simulink model "model_sim_CHB5_36_new_temp"  (R2020a)
settings: Solver=FixedStepAuto  StartTime=0.0  StopTime=5  RelTol=1e-3
InitFcn:
  | sysinit
values from neighbouring files (symbols this model uses):
  C = 0.03    [sysinit.m]
  C_f = 0.625e-6    (= 6.25e-07)    [sysinit.m]
  f = 50    [sysinit.m]
  f_switch = 500    [sysinit.m]
  L = 0.004    [sysinit.m]
  L_f = 3e-6    (= 3e-06)    [sysinit.m]
  R = 1.2    [sysinit.m]
  R_f = 1.5    [sysinit.m]
  Rth_h = 7.5e-3    (= 0.0075)    [Device_Parameter.m]
  Rth_h_tau = 0.5    [Device_Parameter.m]
  st = 5e-7    (= 5e-07)    [sysinit.m]
  temp_init = 40    [sysinit.m]
  Ts = 1e-6    (= 1e-06)    [sysinit.m]
  Ts2 = 0.5E-3    (= 0.0005)    [sysinit.m]
  Udc = 2500    [sysinit.m]
undefined symbols (not defined in the file or in its folder): DIODE_204520, DIODE_344520, DIODE_D1031SH, DIODE_D1331SH, IGCT_364520_36, IGCT_364521_36, IGCT_654522_6, magnitude, Ts1
libraries: powerlib x278, powerlib_meascontrol x84, simulink x9
(part 3 of 5)

== system model_sim_CHB5_36_new_temp/Uref/Saddle_Wave ==
  A : Inport
  B : Inport  Port=2
  C : Inport  Port=3
  Add{1..3,9} (4 alike) : Sum
  Gain : Gain  Gain=-0.5
  Max : MinMax  Function=max  Inputs=3
  Max1 : MinMax  Inputs=3
  a : Outport
  b : Outport  Port=2
  c : Outport  Port=3
  wires:
  B/1 -> Add3/2, Max1/2, Max/2
  C/1 -> Add9/2, Max1/3, Max/3
  A/1 -> Max1/1, Add2/2, Max/1
  Gain/1 -> Add9/1, Add3/1, Add2/1
  Max/1 -> Add1/1
  Max1/1 -> Add1/2
  Add1/1 -> Gain/1
  Add9/1 -> c/1
  Add2/1 -> a/1
  Add3/1 -> b/1

== system model_sim_CHB5_36_new_temp/pwm generator/carrier ==
  Mux : Mux
  Repeating Sequence1 : simulink/Sources/Repeating Sequence  rep_seq_t=[0 0.5 1]/f_car  rep_seq_y=[-1 1 -1]*1000
  Scope1 : Scope  NumInputPorts=4
  Transport Delay1 : TransportDelay  DelayTime=tt/f_car  BufferSize=3072
  Transport Delay3 : TransportDelay  DelayTime=tt/f_car  BufferSize=3072
  Transport Delay4 : TransportDelay  DelayTime=tt/f_car  BufferSize=3072
  CARRIER_4*1 : Outport
  wires:
  Repeating Sequence1/1 -> Scope1/1, Mux/1, Transport Delay1/1
  Transport Delay1/1 -> Scope1/2, Mux/2, Transport Delay3/1
  Mux/1 -> CARRIER_4*1/1
  Transport Delay3/1 -> Mux/3, Scope1/3, Transport Delay4/1
  Transport Delay4/1 -> Mux/4, Scope1/4

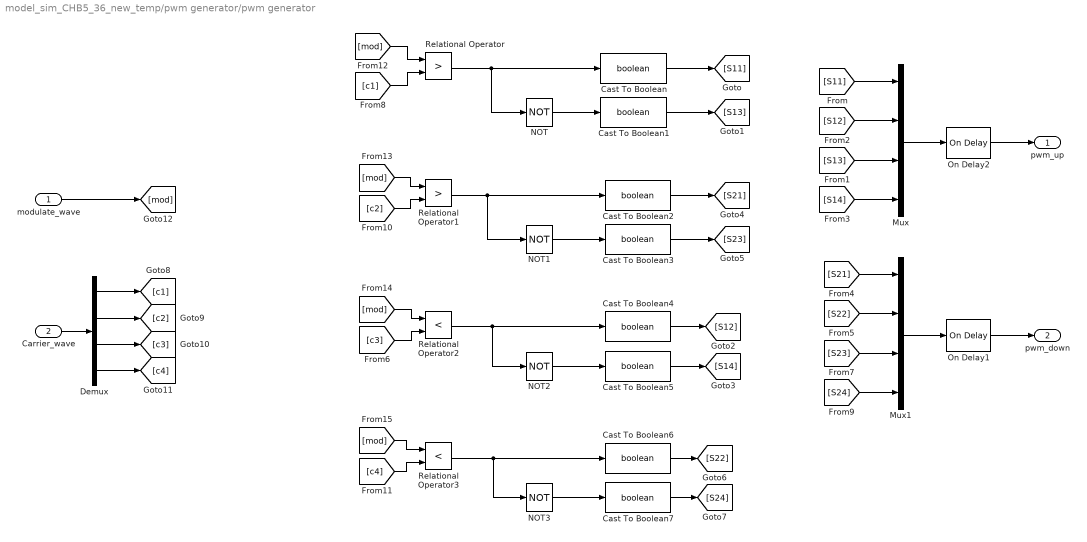
== system model_sim_CHB5_36_new_temp/pwm generator/pwm generator ==
  modulate_wave : Inport
  Carrier_wave : Inport  Port=2
  Cast To Boolean{,1..7} (8 alike) : DataTypeConversion  OutDataTypeStr=boolean
  Demux : Demux
  Mux : Mux
  Mux1 : Mux
  NOT{,1..3} (4 alike) : Logic  Operator=NOT  AllPortsSameDT=off  OutDataTypeStr=boolean
  On Delay1 : powerlib_meascontrol/Logic/On Delay  DelayType=On delay  delay=ttd  ic=0  Ts=0
  On Delay2 : powerlib_meascontrol/Logic/On Delay  DelayType=On delay  delay=ttd  ic=0  Ts=0
  Relational Operator : RelationalOperator  Operator=>  OutDataTypeStr=boolean  RndMeth=Simplest
  Relational Operator1 : RelationalOperator  Operator=>  OutDataTypeStr=boolean  RndMeth=Simplest
  Relational Operator2 : RelationalOperator  Operator=<  OutDataTypeStr=boolean  RndMeth=Simplest
  Relational Operator3 : RelationalOperator  Operator=<  OutDataTypeStr=boolean  RndMeth=Simplest
  pwm_up : Outport
  pwm_down : Outport  Port=2
  wires:
  NOT/1 -> Cast To Boolean1/1
  [S14] -> Mux/4
  [S23] -> Mux1/3
  [S12] -> Mux/2
  NOT2/1 -> Cast To Boolean5/1
  [S21] -> Mux1/1
  Relational Operator1/1 -> NOT1/1, Cast To Boolean2/1
  [S22] -> Mux1/2
  NOT3/1 -> Cast To Boolean7/1
  Mux/1 -> On Delay2/1
  [S24] -> Mux1/4
  [S13] -> Mux/3
  Relational Operator2/1 -> Cast To Boolean4/1, NOT2/1
  [S11] -> Mux/1
  Relational Operator/1 -> NOT/1, Cast To Boolean/1
  NOT1/1 -> Cast To Boolean3/1
  Mux1/1 -> On Delay1/1
  Relational Operator3/1 -> Cast To Boolean6/1, NOT3/1
  On Delay1/1 -> pwm_down/1
  On Delay2/1 -> pwm_up/1
  Cast To Boolean/1 -> [S11]
  Cast To Boolean1/1 -> [S13]
  Cast To Boolean2/1 -> [S21]
  Cast To Boolean3/1 -> [S23]
  Cast To Boolean4/1 -> [S12]
  Cast To Boolean5/1 -> [S14]
  Cast To Boolean6/1 -> [S22]
  Cast To Boolean7/1 -> [S24]
  Carrier_wave/1 -> Demux/1
  Demux/1 -> [c1]
  [c3] -> Relational Operator2/2
  Demux/2 -> [c2]
  Demux/4 -> [c4]
  Demux/3 -> [c3]
  [c1] -> Relational Operator/2
  [c2] -> Relational Operator1/2
  [c4] -> Relational Operator3/2
  modulate_wave/1 -> [mod]
  [mod] -> Relational Operator/1
  [mod] -> Relational Operator3/1
  [mod] -> Relational Operator2/1
  [mod] -> Relational Operator1/1

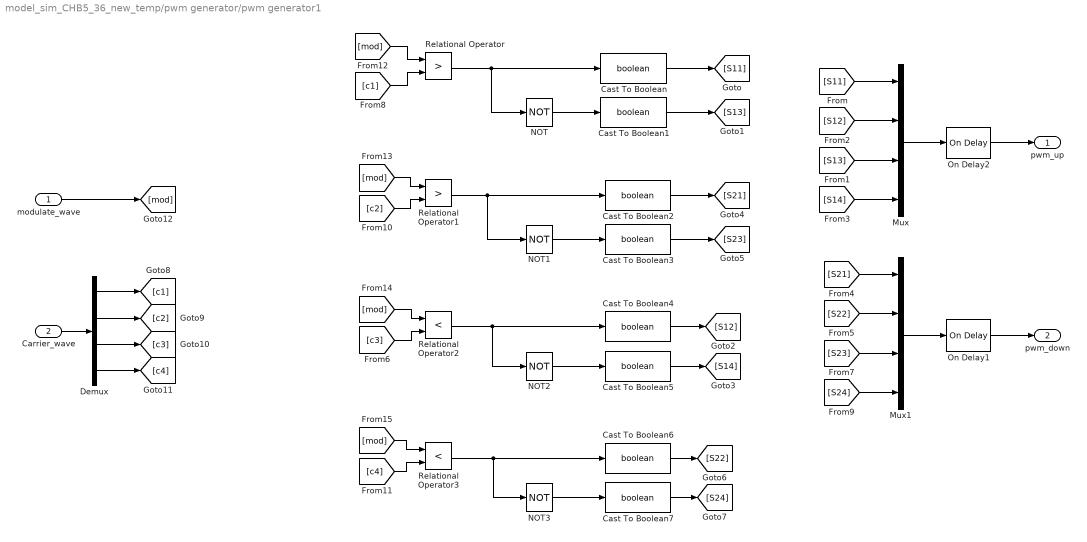
== system model_sim_CHB5_36_new_temp/pwm generator/pwm generator1 ==
  modulate_wave : Inport
  Carrier_wave : Inport  Port=2
  Cast To Boolean{,1..7} (8 alike) : DataTypeConversion  OutDataTypeStr=boolean
  Demux : Demux
  Mux : Mux
  Mux1 : Mux
  NOT{,1..3} (4 alike) : Logic  Operator=NOT  AllPortsSameDT=off  OutDataTypeStr=boolean
  On Delay1 : powerlib_meascontrol/Logic/On Delay  DelayType=On delay  delay=ttd  ic=0  Ts=0
  On Delay2 : powerlib_meascontrol/Logic/On Delay  DelayType=On delay  delay=ttd  ic=0  Ts=0
  Relational Operator : RelationalOperator  Operator=>  OutDataTypeStr=boolean  RndMeth=Simplest
  Relational Operator1 : RelationalOperator  Operator=>  OutDataTypeStr=boolean  RndMeth=Simplest
  Relational Operator2 : RelationalOperator  Operator=<  OutDataTypeStr=boolean  RndMeth=Simplest
  Relational Operator3 : RelationalOperator  Operator=<  OutDataTypeStr=boolean  RndMeth=Simplest
  pwm_up : Outport
  pwm_down : Outport  Port=2
  wires:
  [mod] -> Relational Operator1/1
  [mod] -> Relational Operator2/1
  [mod] -> Relational Operator3/1
  [mod] -> Relational Operator/1
  modulate_wave/1 -> [mod]
  [c4] -> Relational Operator3/2
  [c2] -> Relational Operator1/2
  [c1] -> Relational Operator/2
  Demux/3 -> [c3]
  Demux/4 -> [c4]
  Demux/2 -> [c2]
  [c3] -> Relational Operator2/2
  Demux/1 -> [c1]
  Carrier_wave/1 -> Demux/1
  Cast To Boolean7/1 -> [S24]
  Cast To Boolean6/1 -> [S22]
  Cast To Boolean5/1 -> [S14]
  Cast To Boolean4/1 -> [S12]
  Cast To Boolean3/1 -> [S23]
  Cast To Boolean2/1 -> [S21]
  Cast To Boolean1/1 -> [S13]
  Cast To Boolean/1 -> [S11]
  On Delay2/1 -> pwm_up/1
  On Delay1/1 -> pwm_down/1
  Relational Operator3/1 -> NOT3/1, Cast To Boolean6/1
  Mux1/1 -> On Delay1/1
  NOT1/1 -> Cast To Boolean3/1
  Relational Operator/1 -> Cast To Boolean/1, NOT/1
  [S11] -> Mux/1
  Relational Operator2/1 -> NOT2/1, Cast To Boolean4/1
  [S13] -> Mux/3
  [S24] -> Mux1/4
  Mux/1 -> On Delay2/1
  NOT3/1 -> Cast To Boolean7/1
  [S22] -> Mux1/2
  Relational Operator1/1 -> Cast To Boolean2/1, NOT1/1
  [S21] -> Mux1/1
  NOT2/1 -> Cast To Boolean5/1
  [S12] -> Mux/2
  [S23] -> Mux1/3
  [S14] -> Mux/4
  NOT/1 -> Cast To Boolean1/1

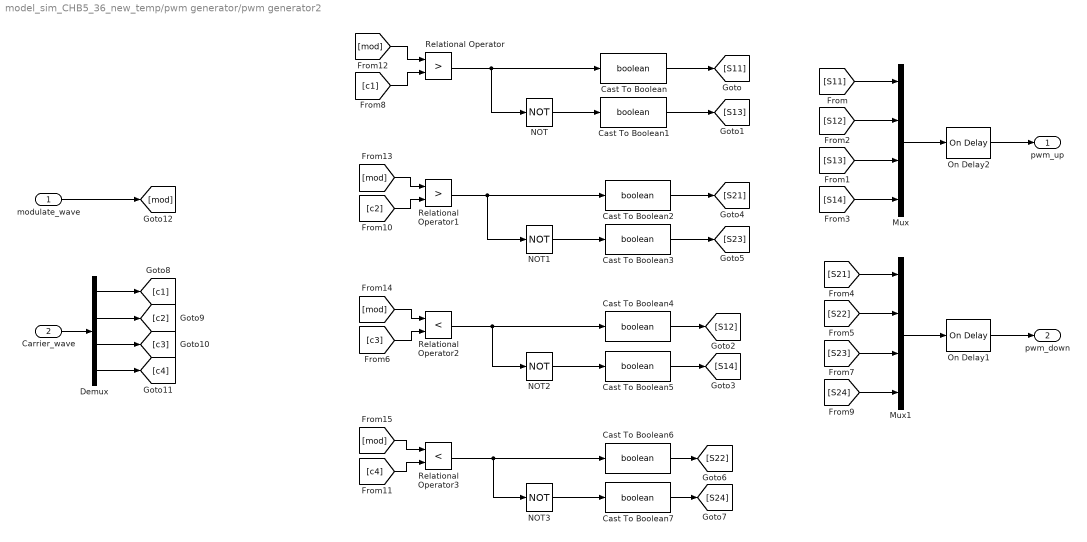
== system model_sim_CHB5_36_new_temp/pwm generator/pwm generator2 ==
  modulate_wave : Inport
  Carrier_wave : Inport  Port=2
  Cast To Boolean{,1..7} (8 alike) : DataTypeConversion  OutDataTypeStr=boolean
  Demux : Demux
  Mux : Mux
  Mux1 : Mux
  NOT{,1..3} (4 alike) : Logic  Operator=NOT  AllPortsSameDT=off  OutDataTypeStr=boolean
  On Delay1 : powerlib_meascontrol/Logic/On Delay  DelayType=On delay  delay=ttd  ic=0  Ts=0
  On Delay2 : powerlib_meascontrol/Logic/On Delay  DelayType=On delay  delay=ttd  ic=0  Ts=0
  Relational Operator : RelationalOperator  Operator=>  OutDataTypeStr=boolean  RndMeth=Simplest
  Relational Operator1 : RelationalOperator  Operator=>  OutDataTypeStr=boolean  RndMeth=Simplest
  Relational Operator2 : RelationalOperator  Operator=<  OutDataTypeStr=boolean  RndMeth=Simplest
  Relational Operator3 : RelationalOperator  Operator=<  OutDataTypeStr=boolean  RndMeth=Simplest
  pwm_up : Outport
  pwm_down : Outport  Port=2
  wires:
  NOT/1 -> Cast To Boolean1/1
  [S14] -> Mux/4
  [S23] -> Mux1/3
  [S12] -> Mux/2
  NOT2/1 -> Cast To Boolean5/1
  [S21] -> Mux1/1
  Relational Operator1/1 -> NOT1/1, Cast To Boolean2/1
  [S22] -> Mux1/2
  NOT3/1 -> Cast To Boolean7/1
  Mux/1 -> On Delay2/1
  [S24] -> Mux1/4
  [S13] -> Mux/3
  Relational Operator2/1 -> Cast To Boolean4/1, NOT2/1
  [S11] -> Mux/1
  Relational Operator/1 -> NOT/1, Cast To Boolean/1
  NOT1/1 -> Cast To Boolean3/1
  Mux1/1 -> On Delay1/1
  Relational Operator3/1 -> Cast To Boolean6/1, NOT3/1
  On Delay1/1 -> pwm_down/1
  On Delay2/1 -> pwm_up/1
  Cast To Boolean/1 -> [S11]
  Cast To Boolean1/1 -> [S13]
  Cast To Boolean2/1 -> [S21]
  Cast To Boolean3/1 -> [S23]
  Cast To Boolean4/1 -> [S12]
  Cast To Boolean5/1 -> [S14]
  Cast To Boolean6/1 -> [S22]
  Cast To Boolean7/1 -> [S24]
  Carrier_wave/1 -> Demux/1
  Demux/1 -> [c1]
  [c3] -> Relational Operator2/2
  Demux/2 -> [c2]
  Demux/4 -> [c4]
  Demux/3 -> [c3]
  [c1] -> Relational Operator/2
  [c2] -> Relational Operator1/2
  [c4] -> Relational Operator3/2
  modulate_wave/1 -> [mod]
  [mod] -> Relational Operator/1
  [mod] -> Relational Operator3/1
  [mod] -> Relational Operator2/1
  [mod] -> Relational Operator1/1

== system model_sim_CHB5_36_new_temp/Subsystem3/DIODE/DIODE_204520 ==
  I : Inport
  PWM1 : Inport  Port=2
  PWM2 : Inport  Port=3
  PWM3 : Inport  Port=4
  PWM4 : Inport  Port=5
  Bus Creator : BusCreator  Inputs=7
  Bus Creator1 : BusCreator  Inputs=7
  Bus Selector : BusSelector  OutputSignals=D1_TEMP,D1_LOSS_MEAN
  Bus Selector1 : BusSelector  OutputSignals=D2_TEMP,D2_LOSS_MEAN
  Constant : Constant
  Constant4 : Constant  Value=0
  Constant5 : Constant
  Constant6 : Constant  Value=0
  Logical Operator : Logic  Operator=OR  AllPortsSameDT=off  OutDataTypeStr=boolean
  Subsystem5 : Subsystem
  Switch : Switch  Criteria=u2 > Threshold  Threshold=DIODE.Junc_temp_lim
  Switch1 : Switch  Criteria=u2 > Threshold  Threshold=DIODE.Junc_temp_lim
  D1_BUS : Outport
  D2_BUS : Outport  Port=2
  D1_LOSS_MEAN : Outport  Port=3
  D2_LOSS_MEAN : Outport  Port=4
  D1_TEMP : Outport  Port=5
  D2_TEMP : Outport  Port=6
  TEMLIM_BOOL : Outport  Port=7
  wires:
  I/1 -> Subsystem5/1(I)
  PWM2/1 -> Subsystem5/3(PWM2)
  PWM3/1 -> Subsystem5/4(PWM3)
  Subsystem5/3(D1_LOSS_MEAN) -> Bus Creator/3
  Subsystem5/12(D2_AVG_MEAN) -> Bus Creator1/5
  Constant6/1 -> Switch1/3
  Subsystem5/14(D2_SW_MEAN) -> Bus Creator1/7
  Switch1/1 -> Logical Operator/2
  Bus Selector1/1 -> Switch1/2, D2_TEMP/1  "<D2_TEMP>"
  Subsystem5/13(D2_SW) -> Bus Creator1/6
  Subsystem5/11(D2_AVG) -> Bus Creator1/4
  Subsystem5/8(D2_TEMP) -> Bus Creator1/1
  Subsystem5/9(D2_LOSS) -> Bus Creator1/2
  Subsystem5/7(D1_SW_MEAN) -> Bus Creator/7
  Switch/1 -> Logical Operator/1
  Constant5/1 -> Switch1/1
  Constant4/1 -> Switch/3
  Subsystem5/1(D1_TEMP) -> Bus Creator/1
  Bus Selector/1 -> Switch/2, D1_TEMP/1  "<D1_TEMP>"
  Subsystem5/6(D1_SW) -> Bus Creator/6
  Bus Creator1/1 -> [D2], D2_BUS/1  "D2_BUS"
  Subsystem5/2(D1_LOSS) -> Bus Creator/2
  Logical Operator/1 -> TEMLIM_BOOL/1
  [D1] -> Bus Selector/1
  Bus Selector/2 -> D1_LOSS_MEAN/1  "<D1_LOSS_MEAN>"
  Subsystem5/5(D1_AVG_MEAN) -> Bus Creator/5
  PWM1/1 -> Subsystem5/2(PWM1)
  PWM4/1 -> Subsystem5/5(PWM4)
  Subsystem5/4(D1_AVG) -> Bus Creator/4
  [D2] -> Bus Selector1/1
  Bus Creator/1 -> [D1], D1_BUS/1  "D1_BUS"
  Bus Selector1/2 -> D2_LOSS_MEAN/1  "<D2_LOSS_MEAN>"
  Subsystem5/10(D2_LOSS_MEAN) -> Bus Creator1/3
  Constant/1 -> Switch/1

== system model_sim_CHB5_36_new_temp/Subsystem3/DIODE/DIODE_344520 ==
  I : Inport
  PWM1 : Inport  Port=2
  PWM2 : Inport  Port=3
  PWM3 : Inport  Port=4
  PWM4 : Inport  Port=5
  Bus Creator : BusCreator  Inputs=7
  Bus Creator1 : BusCreator  Inputs=7
  Bus Selector : BusSelector  OutputSignals=D1_TEMP,D1_LOSS_MEAN
  Bus Selector1 : BusSelector  OutputSignals=D2_TEMP,D2_LOSS_MEAN
  Constant : Constant
  Constant4 : Constant  Value=0
  Constant5 : Constant
  Constant6 : Constant  Value=0
  Logical Operator : Logic  Operator=OR  AllPortsSameDT=off  OutDataTypeStr=boolean
  Subsystem5 : Subsystem
  Switch : Switch  Criteria=u2 > Threshold  Threshold=DIODE.Junc_temp_lim
  Switch1 : Switch  Criteria=u2 > Threshold  Threshold=DIODE.Junc_temp_lim
  D1_BUS : Outport
  D2_BUS : Outport  Port=2
  D1_LOSS_MEAN : Outport  Port=3
  D2_LOSS_MEAN : Outport  Port=4
  D1_TEMP : Outport  Port=5
  D2_TEMP : Outport  Port=6
  TEMLIM_BOOL : Outport  Port=7
  wires:
  Constant/1 -> Switch/1
  Subsystem5/10(D2_LOSS_MEAN) -> Bus Creator1/3
  Bus Selector1/2 -> D2_LOSS_MEAN/1  "<D2_LOSS_MEAN>"
  Bus Creator/1 -> D1_BUS/1, [D1]  "D1_BUS"
  [D2] -> Bus Selector1/1
  Subsystem5/4(D1_AVG) -> Bus Creator/4
  PWM4/1 -> Subsystem5/5(PWM4)
  PWM1/1 -> Subsystem5/2(PWM1)
  Subsystem5/5(D1_AVG_MEAN) -> Bus Creator/5
  Bus Selector/2 -> D1_LOSS_MEAN/1  "<D1_LOSS_MEAN>"
  [D1] -> Bus Selector/1
  Logical Operator/1 -> TEMLIM_BOOL/1
  Subsystem5/2(D1_LOSS) -> Bus Creator/2
  Bus Creator1/1 -> D2_BUS/1, [D2]  "D2_BUS"
  Subsystem5/6(D1_SW) -> Bus Creator/6
  Bus Selector/1 -> D1_TEMP/1, Switch/2  "<D1_TEMP>"
  Subsystem5/1(D1_TEMP) -> Bus Creator/1
  Constant4/1 -> Switch/3
  Constant5/1 -> Switch1/1
  Switch/1 -> Logical Operator/1
  Subsystem5/7(D1_SW_MEAN) -> Bus Creator/7
  Subsystem5/9(D2_LOSS) -> Bus Creator1/2
  Subsystem5/8(D2_TEMP) -> Bus Creator1/1
  Subsystem5/11(D2_AVG) -> Bus Creator1/4
  Subsystem5/13(D2_SW) -> Bus Creator1/6
  Bus Selector1/1 -> D2_TEMP/1, Switch1/2  "<D2_TEMP>"
  Switch1/1 -> Logical Operator/2
  Subsystem5/14(D2_SW_MEAN) -> Bus Creator1/7
  Constant6/1 -> Switch1/3
  Subsystem5/12(D2_AVG_MEAN) -> Bus Creator1/5
  Subsystem5/3(D1_LOSS_MEAN) -> Bus Creator/3
  PWM3/1 -> Subsystem5/4(PWM3)
  PWM2/1 -> Subsystem5/3(PWM2)
  I/1 -> Subsystem5/1(I)

== system model_sim_CHB5_36_new_temp/Subsystem3/DIODE/DIODE_D1031SH ==
  I : Inport
  PWM1 : Inport  Port=2
  PWM2 : Inport  Port=3
  PWM3 : Inport  Port=4
  PWM4 : Inport  Port=5
  Bus Creator : BusCreator  Inputs=7
  Bus Creator1 : BusCreator  Inputs=7
  Bus Selector : BusSelector  OutputSignals=D1_TEMP,D1_LOSS_MEAN
  Bus Selector1 : BusSelector  OutputSignals=D2_TEMP,D2_LOSS_MEAN
  Constant : Constant
  Constant4 : Constant  Value=0
  Constant5 : Constant
  Constant6 : Constant  Value=0
  Logical Operator : Logic  Operator=OR  AllPortsSameDT=off  OutDataTypeStr=boolean
  Subsystem5 : Subsystem
  Switch : Switch  Criteria=u2 > Threshold  Threshold=DIODE.Junc_temp_lim
  Switch1 : Switch  Criteria=u2 > Threshold  Threshold=DIODE.Junc_temp_lim
  D1_BUS : Outport
  D2_BUS : Outport  Port=2
  D1_LOSS_MEAN : Outport  Port=3
  D2_LOSS_MEAN : Outport  Port=4
  D1_TEMP : Outport  Port=5
  D2_TEMP : Outport  Port=6
  TEMLIM_BOOL : Outport  Port=7
  wires:
  I/1 -> Subsystem5/1(I)
  PWM2/1 -> Subsystem5/3(PWM2)
  PWM3/1 -> Subsystem5/4(PWM3)
  Subsystem5/3(D1_LOSS_MEAN) -> Bus Creator/3
  Subsystem5/12(D2_AVG_MEAN) -> Bus Creator1/5
  Constant6/1 -> Switch1/3
  Subsystem5/14(D2_SW_MEAN) -> Bus Creator1/7
  Switch1/1 -> Logical Operator/2
  Bus Selector1/1 -> Switch1/2, D2_TEMP/1  "<D2_TEMP>"
  Subsystem5/13(D2_SW) -> Bus Creator1/6
  Subsystem5/11(D2_AVG) -> Bus Creator1/4
  Subsystem5/8(D2_TEMP) -> Bus Creator1/1
  Subsystem5/9(D2_LOSS) -> Bus Creator1/2
  Subsystem5/7(D1_SW_MEAN) -> Bus Creator/7
  Switch/1 -> Logical Operator/1
  Constant5/1 -> Switch1/1
  Constant4/1 -> Switch/3
  Subsystem5/1(D1_TEMP) -> Bus Creator/1
  Bus Selector/1 -> Switch/2, D1_TEMP/1  "<D1_TEMP>"
  Subsystem5/6(D1_SW) -> Bus Creator/6
  Bus Creator1/1 -> [D2], D2_BUS/1  "D2_BUS"
  Subsystem5/2(D1_LOSS) -> Bus Creator/2
  Logical Operator/1 -> TEMLIM_BOOL/1
  [D1] -> Bus Selector/1
  Bus Selector/2 -> D1_LOSS_MEAN/1  "<D1_LOSS_MEAN>"
  Subsystem5/5(D1_AVG_MEAN) -> Bus Creator/5
  PWM1/1 -> Subsystem5/2(PWM1)
  PWM4/1 -> Subsystem5/5(PWM4)
  Subsystem5/4(D1_AVG) -> Bus Creator/4
  [D2] -> Bus Selector1/1
  Bus Creator/1 -> [D1], D1_BUS/1  "D1_BUS"
  Bus Selector1/2 -> D2_LOSS_MEAN/1  "<D2_LOSS_MEAN>"
  Subsystem5/10(D2_LOSS_MEAN) -> Bus Creator1/3
  Constant/1 -> Switch/1

== system model_sim_CHB5_36_new_temp/Subsystem3/DIODE/DIODE_D1331SH ==
  I : Inport
  PWM1 : Inport  Port=2
  PWM2 : Inport  Port=3
  PWM3 : Inport  Port=4
  PWM4 : Inport  Port=5
  Bus Creator : BusCreator  Inputs=7
  Bus Creator1 : BusCreator  Inputs=7
  Bus Selector : BusSelector  OutputSignals=D1_TEMP,D1_LOSS_MEAN
  Bus Selector1 : BusSelector  OutputSignals=D2_TEMP,D2_LOSS_MEAN
  Constant : Constant
  Constant4 : Constant  Value=0
  Constant5 : Constant
  Constant6 : Constant  Value=0
  Logical Operator : Logic  Operator=OR  AllPortsSameDT=off  OutDataTypeStr=boolean
  Subsystem5 : Subsystem
  Switch : Switch  Criteria=u2 > Threshold  Threshold=DIODE.Junc_temp_lim
  Switch1 : Switch  Criteria=u2 > Threshold  Threshold=DIODE.Junc_temp_lim
  D1_BUS : Outport
  D2_BUS : Outport  Port=2
  D1_LOSS_MEAN : Outport  Port=3
  D2_LOSS_MEAN : Outport  Port=4
  D1_TEMP : Outport  Port=5
  D2_TEMP : Outport  Port=6
  TEMLIM_BOOL : Outport  Port=7
  wires:
  Constant/1 -> Switch/1
  Subsystem5/10(D2_LOSS_MEAN) -> Bus Creator1/3
  Bus Selector1/2 -> D2_LOSS_MEAN/1  "<D2_LOSS_MEAN>"
  Bus Creator/1 -> D1_BUS/1, [D1]  "D1_BUS"
  [D2] -> Bus Selector1/1
  Subsystem5/4(D1_AVG) -> Bus Creator/4
  PWM4/1 -> Subsystem5/5(PWM4)
  PWM1/1 -> Subsystem5/2(PWM1)
  Subsystem5/5(D1_AVG_MEAN) -> Bus Creator/5
  Bus Selector/2 -> D1_LOSS_MEAN/1  "<D1_LOSS_MEAN>"
  [D1] -> Bus Selector/1
  Logical Operator/1 -> TEMLIM_BOOL/1
  Subsystem5/2(D1_LOSS) -> Bus Creator/2
  Bus Creator1/1 -> D2_BUS/1, [D2]  "D2_BUS"
  Subsystem5/6(D1_SW) -> Bus Creator/6
  Bus Selector/1 -> D1_TEMP/1, Switch/2  "<D1_TEMP>"
  Subsystem5/1(D1_TEMP) -> Bus Creator/1
  Constant4/1 -> Switch/3
  Constant5/1 -> Switch1/1
  Switch/1 -> Logical Operator/1
  Subsystem5/7(D1_SW_MEAN) -> Bus Creator/7
  Subsystem5/9(D2_LOSS) -> Bus Creator1/2
  Subsystem5/8(D2_TEMP) -> Bus Creator1/1
  Subsystem5/11(D2_AVG) -> Bus Creator1/4
  Subsystem5/13(D2_SW) -> Bus Creator1/6
  Bus Selector1/1 -> D2_TEMP/1, Switch1/2  "<D2_TEMP>"
  Switch1/1 -> Logical Operator/2
  Subsystem5/14(D2_SW_MEAN) -> Bus Creator1/7
  Constant6/1 -> Switch1/3
  Subsystem5/12(D2_AVG_MEAN) -> Bus Creator1/5
  Subsystem5/3(D1_LOSS_MEAN) -> Bus Creator/3
  PWM3/1 -> Subsystem5/4(PWM3)
  PWM2/1 -> Subsystem5/3(PWM2)
  I/1 -> Subsystem5/1(I)

== system model_sim_CHB5_36_new_temp/Subsystem3/IGCT/IGCT_364520_36 ==
  I : Inport
  PWM1 : Inport  Port=2
  PWM2 : Inport  Port=3
  Bus Creator : BusCreator  Inputs=7
  Bus Creator1 : BusCreator  Inputs=7
  Bus Selector : BusSelector  OutputSignals=T1_TEMP,T1_LOSS_MEAN
  Bus Selector1 : BusSelector  OutputSignals=T2_TEMP,T2_LOSS_MEAN
  Constant : Constant
  Constant10 : Constant
  Constant11 : Constant  Value=0
  Constant9 : Constant  Value=0
  Logical Operator2 : Logic  Operator=OR  AllPortsSameDT=off  OutDataTypeStr=boolean
  MAIN : Subsystem
  Switch4 : Switch  Criteria=u2 > Threshold  Threshold=IGCT.Junc_temp_lim
  Switch5 : Switch  Criteria=u2 > Threshold  Threshold=IGCT.Junc_temp_lim
  T1_BUS : Outport
  T2_BUS : Outport  Port=2
  <T1_TEMP> : Outport  Port=3
  <T2_TEMP> : Outport  Port=4
  <T1_LOSS_MEAN> : Outport  Port=5
  <T2_LOSS_MEAN> : Outport  Port=6
  TEMLIM_BOOL : Outport  Port=7
  wires:
  MAIN/7(T1_SW_MEAN) -> Bus Creator/7  "T1_SW_MEAN"
  I/1 -> MAIN/1(I)
  MAIN/9(T2_LOSS) -> Bus Creator1/2  "T2_LOSS"
  PWM2/1 -> MAIN/3(T2)
  Logical Operator2/1 -> TEMLIM_BOOL/1
  MAIN/2(T1_LOSS) -> Bus Creator/2  "T1_LOSS"
  MAIN/8(T2_TEMP) -> Bus Creator1/1  "T2_TEMP"
  [T2] -> Bus Selector1/1
  Bus Selector/2 -> <T1_LOSS_MEAN>/1  "<T1_LOSS_MEAN>"
  MAIN/11(T2_AVG) -> Bus Creator1/4  "T2_AVG"
  PWM1/1 -> MAIN/2(T1)
  Bus Selector1/2 -> <T2_LOSS_MEAN>/1  "<T2_LOSS_MEAN>"
  Constant9/1 -> Switch4/3
  Switch4/1 -> Logical Operator2/1
  MAIN/4(T1_AVG) -> Bus Creator/4  "T1_AVG"
  Bus Creator1/1 -> [T2], T2_BUS/1
  Bus Selector/1 -> Switch4/2, <T1_TEMP>/1  "<T1_TEMP>"
  MAIN/6(T1_SW) -> Bus Creator/6  "T1_SW"
  Constant/1 -> Switch4/1
  Bus Creator/1 -> [T1], T1_BUS/1
  MAIN/12(T2_AVG_MEAN) -> Bus Creator1/5  "T2_AVG_MEAN"
  MAIN/5(T1_AVG_MEAN) -> Bus Creator/5  "T1_AVG_MEAN"
  Constant10/1 -> Switch5/1
  Constant11/1 -> Switch5/3
  MAIN/13(T2_SW) -> Bus Creator1/6  "T2_SW"
  MAIN/3(T1_LOSS_MEAN) -> Bus Creator/3  "T1_LOSS_MEAN"
  Bus Selector1/1 -> Switch5/2, <T2_TEMP>/1  "<T2_TEMP>"
  MAIN/10(T2_LOSS_MEAN) -> Bus Creator1/3  "T2_LOSS_MEAN"
  MAIN/14(T2_SW_MEAN) -> Bus Creator1/7  "T2_SW_MEAN"
  MAIN/1(T1_TEMP) -> Bus Creator/1  "T1_TEMP"
  [T1] -> Bus Selector/1
  Switch5/1 -> Logical Operator2/2

== system model_sim_CHB5_36_new_temp/Subsystem3/IGCT/IGCT_364521_36 ==
  I : Inport
  PWM1 : Inport  Port=2
  PWM2 : Inport  Port=3
  Bus Creator : BusCreator  Inputs=7
  Bus Creator1 : BusCreator  Inputs=7
  Bus Selector : BusSelector  OutputSignals=T1_TEMP,T1_LOSS_MEAN
  Bus Selector1 : BusSelector  OutputSignals=T2_TEMP,T2_LOSS_MEAN
  Constant : Constant
  Constant10 : Constant
  Constant11 : Constant  Value=0
  Constant9 : Constant  Value=0
  Logical Operator2 : Logic  Operator=OR  AllPortsSameDT=off  OutDataTypeStr=boolean
  MAIN : Subsystem
  Switch4 : Switch  Criteria=u2 > Threshold  Threshold=IGCT.Junc_temp_lim
  Switch5 : Switch  Criteria=u2 > Threshold  Threshold=IGCT.Junc_temp_lim
  T1_BUS : Outport
  T2_BUS : Outport  Port=2
  <T1_TEMP> : Outport  Port=3
  <T2_TEMP> : Outport  Port=4
  <T1_LOSS_MEAN> : Outport  Port=5
  <T2_LOSS_MEAN> : Outport  Port=6
  TEMLIM_BOOL : Outport  Port=7
  wires:
  Switch5/1 -> Logical Operator2/2
  [T1] -> Bus Selector/1
  MAIN/1(T1_TEMP) -> Bus Creator/1  "T1_TEMP"
  MAIN/14(T2_SW_MEAN) -> Bus Creator1/7  "T2_SW_MEAN"
  MAIN/10(T2_LOSS_MEAN) -> Bus Creator1/3  "T2_LOSS_MEAN"
  Bus Selector1/1 -> <T2_TEMP>/1, Switch5/2  "<T2_TEMP>"
  MAIN/3(T1_LOSS_MEAN) -> Bus Creator/3  "T1_LOSS_MEAN"
  MAIN/13(T2_SW) -> Bus Creator1/6  "T2_SW"
  Constant11/1 -> Switch5/3
  Constant10/1 -> Switch5/1
  MAIN/5(T1_AVG_MEAN) -> Bus Creator/5  "T1_AVG_MEAN"
  MAIN/12(T2_AVG_MEAN) -> Bus Creator1/5  "T2_AVG_MEAN"
  Bus Creator/1 -> T1_BUS/1, [T1]
  Constant/1 -> Switch4/1
  MAIN/6(T1_SW) -> Bus Creator/6  "T1_SW"
  Bus Selector/1 -> <T1_TEMP>/1, Switch4/2  "<T1_TEMP>"
  Bus Creator1/1 -> T2_BUS/1, [T2]
  MAIN/4(T1_AVG) -> Bus Creator/4  "T1_AVG"
  Switch4/1 -> Logical Operator2/1
  Constant9/1 -> Switch4/3
  Bus Selector1/2 -> <T2_LOSS_MEAN>/1  "<T2_LOSS_MEAN>"
  PWM1/1 -> MAIN/2(T1)
  MAIN/11(T2_AVG) -> Bus Creator1/4  "T2_AVG"
  Bus Selector/2 -> <T1_LOSS_MEAN>/1  "<T1_LOSS_MEAN>"
  [T2] -> Bus Selector1/1
  MAIN/8(T2_TEMP) -> Bus Creator1/1  "T2_TEMP"
  MAIN/2(T1_LOSS) -> Bus Creator/2  "T1_LOSS"
  Logical Operator2/1 -> TEMLIM_BOOL/1
  PWM2/1 -> MAIN/3(T2)
  MAIN/9(T2_LOSS) -> Bus Creator1/2  "T2_LOSS"
  I/1 -> MAIN/1(I)
  MAIN/7(T1_SW_MEAN) -> Bus Creator/7  "T1_SW_MEAN"

== system model_sim_CHB5_36_new_temp/Subsystem3/IGCT/IGCT_654522_6 ==
  I : Inport
  PWM1 : Inport  Port=2
  PWM2 : Inport  Port=3
  Bus Creator : BusCreator  Inputs=7
  Bus Creator1 : BusCreator  Inputs=7
  Bus Selector : BusSelector  OutputSignals=T1_TEMP,T1_LOSS_MEAN
  Bus Selector1 : BusSelector  OutputSignals=T2_TEMP,T2_LOSS_MEAN
  Constant : Constant
  Constant10 : Constant
  Constant11 : Constant  Value=0
  Constant9 : Constant  Value=0
  Logical Operator2 : Logic  Operator=OR  AllPortsSameDT=off  OutDataTypeStr=boolean
  MAIN : Subsystem
  Switch4 : Switch  Criteria=u2 > Threshold  Threshold=IGCT.Junc_temp_lim
  Switch5 : Switch  Criteria=u2 > Threshold  Threshold=IGCT.Junc_temp_lim
  T1_BUS : Outport
  T2_BUS : Outport  Port=2
  <T1_TEMP> : Outport  Port=3
  <T2_TEMP> : Outport  Port=4
  <T1_LOSS_MEAN> : Outport  Port=5
  <T2_LOSS_MEAN> : Outport  Port=6
  TEMLIM_BOOL : Outport  Port=7
  wires:
  Switch5/1 -> Logical Operator2/2
  [T1] -> Bus Selector/1
  MAIN/1(T1_TEMP) -> Bus Creator/1  "T1_TEMP"
  MAIN/14(T2_SW_MEAN) -> Bus Creator1/7  "T2_SW_MEAN"
  MAIN/10(T2_LOSS_MEAN) -> Bus Creator1/3  "T2_LOSS_MEAN"
  Bus Selector1/1 -> <T2_TEMP>/1, Switch5/2  "<T2_TEMP>"
  MAIN/3(T1_LOSS_MEAN) -> Bus Creator/3  "T1_LOSS_MEAN"
  MAIN/13(T2_SW) -> Bus Creator1/6  "T2_SW"
  Constant11/1 -> Switch5/3
  Constant10/1 -> Switch5/1
  MAIN/5(T1_AVG_MEAN) -> Bus Creator/5  "T1_AVG_MEAN"
  MAIN/12(T2_AVG_MEAN) -> Bus Creator1/5  "T2_AVG_MEAN"
  Bus Creator/1 -> T1_BUS/1, [T1]
  Constant/1 -> Switch4/1
  MAIN/6(T1_SW) -> Bus Creator/6  "T1_SW"
  Bus Selector/1 -> <T1_TEMP>/1, Switch4/2  "<T1_TEMP>"
  Bus Creator1/1 -> T2_BUS/1, [T2]
  MAIN/4(T1_AVG) -> Bus Creator/4  "T1_AVG"
  Switch4/1 -> Logical Operator2/1
  Constant9/1 -> Switch4/3
  Bus Selector1/2 -> <T2_LOSS_MEAN>/1  "<T2_LOSS_MEAN>"
  PWM1/1 -> MAIN/2(T1)
  MAIN/11(T2_AVG) -> Bus Creator1/4  "T2_AVG"
  Bus Selector/2 -> <T1_LOSS_MEAN>/1  "<T1_LOSS_MEAN>"
  [T2] -> Bus Selector1/1
  MAIN/8(T2_TEMP) -> Bus Creator1/1  "T2_TEMP"
  MAIN/2(T1_LOSS) -> Bus Creator/2  "T1_LOSS"
  Logical Operator2/1 -> TEMLIM_BOOL/1
  PWM2/1 -> MAIN/3(T2)
  MAIN/9(T2_LOSS) -> Bus Creator1/2  "T2_LOSS"
  I/1 -> MAIN/1(I)
  MAIN/7(T1_SW_MEAN) -> Bus Creator/7  "T1_SW_MEAN"

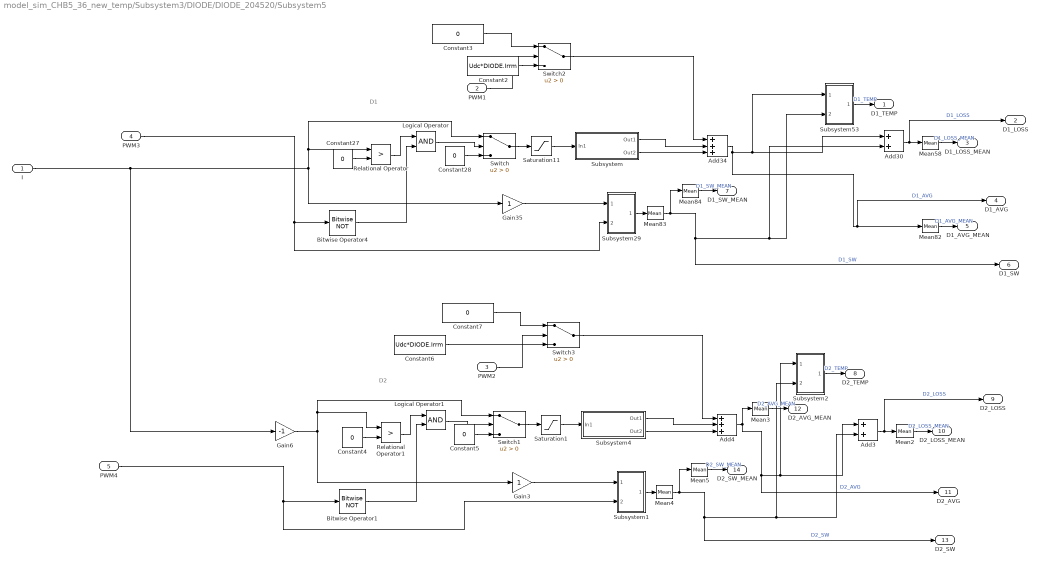
== system model_sim_CHB5_36_new_temp/Subsystem3/DIODE/DIODE_204520/Subsystem5 ==
  note: D2
  note: D1
  I : Inport
  PWM1 : Inport  Port=2
  PWM2 : Inport  Port=3
  PWM3 : Inport  Port=4
  PWM4 : Inport  Port=5
  Add3 : Sum
  Add30 : Sum
  Add34 : Sum  Inputs=+++
  Add4 : Sum  Inputs=+++
  Bitwise Operator1 : simulink/Logic and Bit Operations/Bitwise Operator  logicop=NOT  UseBitMask=off  BitMask=bin2dec('11011001')  BitMaskRealWorld=Stored Integer
  Bitwise Operator4 : simulink/Logic and Bit Operations/Bitwise Operator  logicop=NOT  UseBitMask=off  BitMask=bin2dec('11011001')  BitMaskRealWorld=Stored Integer
  Constant2 : Constant  Value=Udc*DIODE.Irrm
  Constant{3..5,7,27..28} (6 alike) : Constant  Value=0
  Constant6 : Constant  Value=Udc*DIODE.Irrm
  Gain3 : Gain
  Gain35 : Gain
  Gain6 : Gain  Gain=-1
  Logical Operator : Logic  AllPortsSameDT=off  OutDataTypeStr=boolean
  Logical Operator1 : Logic  AllPortsSameDT=off  OutDataTypeStr=boolean
  Mean{2..3,5,58,82,84} (6 alike) : powerlib_meascontrol/Measurements/Mean  Freq=f  Vinit=0  Ts=1e-6
  Mean4 : powerlib_meascontrol/Measurements/Mean  Freq=2000  Vinit=0  Ts=1e-6
  Mean83 : powerlib_meascontrol/Measurements/Mean  Freq=2000  Vinit=0  Ts=1e-6
  Relational Operator : RelationalOperator  Operator=>  OutDataTypeStr=boolean  RndMeth=Simplest
  Relational Operator1 : RelationalOperator  Operator=>  OutDataTypeStr=boolean  RndMeth=Simplest
  Saturation1 : Saturate  UpperLimit=5500  LowerLimit=0
  Saturation11 : Saturate  UpperLimit=5500  LowerLimit=0
  Subsystem : Subsystem
  Subsystem1 : Subsystem
  Subsystem2 : Subsystem
  Subsystem29 : Subsystem
  Subsystem4 : Subsystem
  Subsystem53 : Subsystem
  Switch{,1..3} (4 alike) : Switch  Criteria=u2 > Threshold
  D1_TEMP : Outport
  D1_LOSS : Outport  Port=2
  D1_LOSS_MEAN : Outport  Port=3
  D1_AVG : Outport  Port=4
  D1_AVG_MEAN : Outport  Port=5
  D1_SW : Outport  Port=6
  D1_SW_MEAN : Outport  Port=7
  D2_TEMP : Outport  Port=8
  D2_LOSS : Outport  Port=9
  D2_LOSS_MEAN : Outport  Port=10
  D2_AVG : Outport  Port=11
  D2_AVG_MEAN : Outport  Port=12
  D2_SW : Outport  Port=13
  D2_SW_MEAN : Outport  Port=14
  wires:
  Mean5/1 -> D2_SW_MEAN/1  "D2_SW_MEAN"
  Subsystem2/1(Out1) -> D2_TEMP/1  "D2_TEMP"
  Mean58/1 -> D1_LOSS_MEAN/1  "D1_LOSS_MEAN"
  PWM1/1 -> Switch2/2
  Mean84/1 -> D1_SW_MEAN/1  "D1_SW_MEAN"
  Saturation1/1 -> Subsystem4/1(In1)
  Subsystem4/1(Out1) -> Add4/2
  Gain3/1 -> Subsystem1/1(In1)
  Mean3/1 -> D2_AVG_MEAN/1  "D2_AVG_MEAN"
  Subsystem1/1(Out1) -> Mean4/1
  Constant6/1 -> Switch3/3
  Constant2/1 -> Switch2/3
  Switch2/1 -> Add34/1
  Constant28/1 -> Switch/3
  Bitwise Operator4/1 -> Logical Operator/2
  Add3/1 -> Mean2/1, D2_LOSS/1  "D2_LOSS"
  Constant3/1 -> Switch2/1
  Constant27/1 -> Relational Operator/2
  Constant7/1 -> Switch3/1
  PWM2/1 -> Switch3/2
  Subsystem/2(Out2) -> Add34/3
  Mean82/1 -> D1_AVG_MEAN/1  "D1_AVG_MEAN"
  Mean4/1 -> Mean5/1, Add3/2, Subsystem2/2(In2), D2_SW/1  "D2_SW"
  Bitwise Operator1/1 -> Logical Operator1/2
  PWM3/1 -> Bitwise Operator4/1, Subsystem29/2(In2)
  Gain6/1 -> Gain3/1, Switch1/1, Relational Operator1/1
  Subsystem29/1(Out1) -> Mean83/1
  Relational Operator1/1 -> Logical Operator1/1
  Relational Operator/1 -> Logical Operator/1
  Switch3/1 -> Add4/1
  Add4/1 -> Subsystem2/1(In1), Add3/1, D2_AVG/1, Mean3/1  "D2_AVG"
  Switch1/1 -> Saturation1/1
  Constant5/1 -> Switch1/3
  Mean83/1 -> Add30/2, Subsystem53/2(In2), D1_SW/1, Mean84/1  "D1_SW"
  Add34/1 -> Mean82/1, D1_AVG/1, Subsystem53/1(In1), Add30/1  "D1_AVG"
  Subsystem53/1(Out1) -> D1_TEMP/1  "D1_TEMP"
  Gain35/1 -> Subsystem29/1(In1)
  Logical Operator/1 -> Switch/2
  Add30/1 -> Mean58/1, D1_LOSS/1  "D1_LOSS"
  Subsystem/1(Out1) -> Add34/2
  Switch/1 -> Saturation11/1
  Constant4/1 -> Relational Operator1/2
  I/1 -> Gain6/1, Gain35/1, Relational Operator/1, Switch/1
  PWM4/1 -> Bitwise Operator1/1, Subsystem1/2(In2)
  Saturation11/1 -> Subsystem/1(In1)
  Mean2/1 -> D2_LOSS_MEAN/1  "D2_LOSS_MEAN"
  Logical Operator1/1 -> Switch1/2
  Subsystem4/2(Out2) -> Add4/3

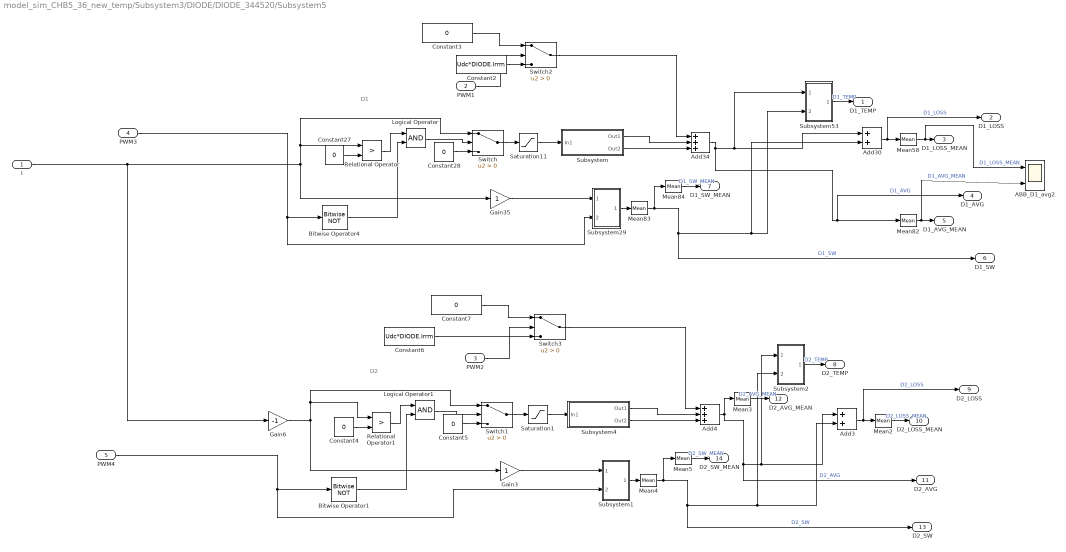
== system model_sim_CHB5_36_new_temp/Subsystem3/DIODE/DIODE_344520/Subsystem5 ==
  note: D1
  note: D2
  I : Inport
  PWM1 : Inport  Port=2
  PWM2 : Inport  Port=3
  PWM3 : Inport  Port=4
  PWM4 : Inport  Port=5
  ABB_D1_avg2 : Scope  NumInputPorts=2
  Add3 : Sum
  Add30 : Sum
  Add34 : Sum  Inputs=+++
  Add4 : Sum  Inputs=+++
  Bitwise Operator1 : simulink/Logic and Bit Operations/Bitwise Operator  logicop=NOT  UseBitMask=off  BitMask=bin2dec('11011001')  BitMaskRealWorld=Stored Integer
  Bitwise Operator4 : simulink/Logic and Bit Operations/Bitwise Operator  logicop=NOT  UseBitMask=off  BitMask=bin2dec('11011001')  BitMaskRealWorld=Stored Integer
  Constant2 : Constant  Value=Udc*DIODE.Irrm
  Constant{3..5,7,27..28} (6 alike) : Constant  Value=0
  Constant6 : Constant  Value=Udc*DIODE.Irrm
  Gain3 : Gain
  Gain35 : Gain
  Gain6 : Gain  Gain=-1
  Logical Operator : Logic  AllPortsSameDT=off  OutDataTypeStr=boolean
  Logical Operator1 : Logic  AllPortsSameDT=off  OutDataTypeStr=boolean
  Mean{2..3,5,58,82,84} (6 alike) : powerlib_meascontrol/Measurements/Mean  Freq=f  Vinit=0  Ts=1e-6
  Mean4 : powerlib_meascontrol/Measurements/Mean  Freq=2000  Vinit=0  Ts=1e-6
  Mean83 : powerlib_meascontrol/Measurements/Mean  Freq=2000  Vinit=0  Ts=1e-6
  Relational Operator : RelationalOperator  Operator=>  OutDataTypeStr=boolean  RndMeth=Simplest
  Relational Operator1 : RelationalOperator  Operator=>  OutDataTypeStr=boolean  RndMeth=Simplest
  Saturation1 : Saturate  UpperLimit=5500  LowerLimit=0
  Saturation11 : Saturate  UpperLimit=5500  LowerLimit=0
  Subsystem : Subsystem
  Subsystem1 : Subsystem
  Subsystem2 : Subsystem
  Subsystem29 : Subsystem
  Subsystem4 : Subsystem
  Subsystem53 : Subsystem
  Switch{,1..3} (4 alike) : Switch  Criteria=u2 > Threshold
  D1_TEMP : Outport
  D1_LOSS : Outport  Port=2
  D1_LOSS_MEAN : Outport  Port=3
  D1_AVG : Outport  Port=4
  D1_AVG_MEAN : Outport  Port=5
  D1_SW : Outport  Port=6
  D1_SW_MEAN : Outport  Port=7
  D2_TEMP : Outport  Port=8
  D2_LOSS : Outport  Port=9
  D2_LOSS_MEAN : Outport  Port=10
  D2_AVG : Outport  Port=11
  D2_AVG_MEAN : Outport  Port=12
  D2_SW : Outport  Port=13
  D2_SW_MEAN : Outport  Port=14
  wires:
  Subsystem4/2(Out2) -> Add4/3
  Logical Operator1/1 -> Switch1/2
  Mean2/1 -> D2_LOSS_MEAN/1  "D2_LOSS_MEAN"
  Saturation11/1 -> Subsystem/1(In1)
  PWM4/1 -> Subsystem1/2(In2), Bitwise Operator1/1
  I/1 -> Switch/1, Relational Operator/1, Gain35/1, Gain6/1
  Constant4/1 -> Relational Operator1/2
  Switch/1 -> Saturation11/1
  Subsystem/1(Out1) -> Add34/2
  Add30/1 -> D1_LOSS/1, Mean58/1  "D1_LOSS"
  Logical Operator/1 -> Switch/2
  Gain35/1 -> Subsystem29/1(In1)
  Subsystem53/1(Out1) -> D1_TEMP/1  "D1_TEMP"
  Add34/1 -> Add30/1, Subsystem53/1(In1), D1_AVG/1, Mean82/1  "D1_AVG"
  Mean83/1 -> Mean84/1, D1_SW/1, Subsystem53/2(In2), Add30/2  "D1_SW"
  Constant5/1 -> Switch1/3
  Switch1/1 -> Saturation1/1
  Add4/1 -> Mean3/1, D2_AVG/1, Add3/1, Subsystem2/1(In1)  "D2_AVG"
  Switch3/1 -> Add4/1
  Relational Operator/1 -> Logical Operator/1
  Relational Operator1/1 -> Logical Operator1/1
  Subsystem29/1(Out1) -> Mean83/1
  Gain6/1 -> Relational Operator1/1, Switch1/1, Gain3/1
  PWM3/1 -> Subsystem29/2(In2), Bitwise Operator4/1
  Bitwise Operator1/1 -> Logical Operator1/2
  Mean4/1 -> D2_SW/1, Subsystem2/2(In2), Add3/2, Mean5/1  "D2_SW"
  Mean82/1 -> ABB_D1_avg2/2, D1_AVG_MEAN/1  "D1_AVG_MEAN"
  Subsystem/2(Out2) -> Add34/3
  PWM2/1 -> Switch3/2
  Constant7/1 -> Switch3/1
  Constant27/1 -> Relational Operator/2
  Constant3/1 -> Switch2/1
  Add3/1 -> D2_LOSS/1, Mean2/1  "D2_LOSS"
  Bitwise Operator4/1 -> Logical Operator/2
  Constant28/1 -> Switch/3
  Switch2/1 -> Add34/1
  Constant2/1 -> Switch2/3
  Constant6/1 -> Switch3/3
  Subsystem1/1(Out1) -> Mean4/1
  Mean3/1 -> D2_AVG_MEAN/1  "D2_AVG_MEAN"
  Gain3/1 -> Subsystem1/1(In1)
  Subsystem4/1(Out1) -> Add4/2
  Saturation1/1 -> Subsystem4/1(In1)
  Mean84/1 -> D1_SW_MEAN/1  "D1_SW_MEAN"
  PWM1/1 -> Switch2/2
  Mean58/1 -> ABB_D1_avg2/1, D1_LOSS_MEAN/1  "D1_LOSS_MEAN"
  Subsystem2/1(Out1) -> D2_TEMP/1  "D2_TEMP"
  Mean5/1 -> D2_SW_MEAN/1  "D2_SW_MEAN"

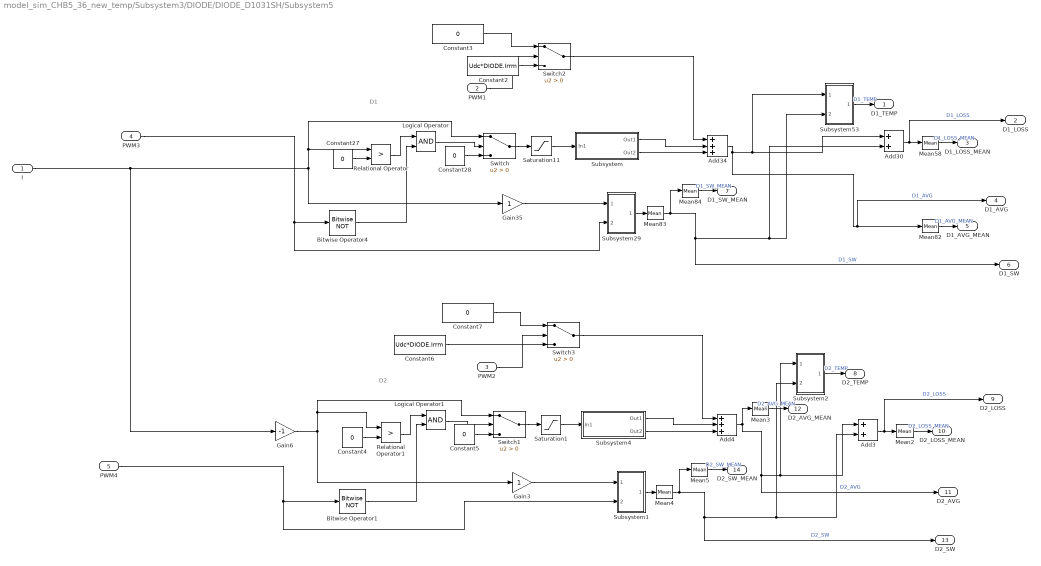
== system model_sim_CHB5_36_new_temp/Subsystem3/DIODE/DIODE_D1031SH/Subsystem5 ==
  note: D2
  note: D1
  I : Inport
  PWM1 : Inport  Port=2
  PWM2 : Inport  Port=3
  PWM3 : Inport  Port=4
  PWM4 : Inport  Port=5
  Add3 : Sum
  Add30 : Sum
  Add34 : Sum  Inputs=+++
  Add4 : Sum  Inputs=+++
  Bitwise Operator1 : simulink/Logic and Bit Operations/Bitwise Operator  logicop=NOT  UseBitMask=off  BitMask=bin2dec('11011001')  BitMaskRealWorld=Stored Integer
  Bitwise Operator4 : simulink/Logic and Bit Operations/Bitwise Operator  logicop=NOT  UseBitMask=off  BitMask=bin2dec('11011001')  BitMaskRealWorld=Stored Integer
  Constant2 : Constant  Value=Udc*DIODE.Irrm
  Constant{3..5,7,27..28} (6 alike) : Constant  Value=0
  Constant6 : Constant  Value=Udc*DIODE.Irrm
  Gain3 : Gain
  Gain35 : Gain
  Gain6 : Gain  Gain=-1
  Logical Operator : Logic  AllPortsSameDT=off  OutDataTypeStr=boolean
  Logical Operator1 : Logic  AllPortsSameDT=off  OutDataTypeStr=boolean
  Mean{2..3,5,58,82,84} (6 alike) : powerlib_meascontrol/Measurements/Mean  Freq=f  Vinit=0  Ts=1e-6
  Mean4 : powerlib_meascontrol/Measurements/Mean  Freq=2000  Vinit=0  Ts=1e-6
  Mean83 : powerlib_meascontrol/Measurements/Mean  Freq=2000  Vinit=0  Ts=1e-6
  Relational Operator : RelationalOperator  Operator=>  OutDataTypeStr=boolean  RndMeth=Simplest
  Relational Operator1 : RelationalOperator  Operator=>  OutDataTypeStr=boolean  RndMeth=Simplest
  Saturation1 : Saturate  UpperLimit=5500  LowerLimit=0
  Saturation11 : Saturate  UpperLimit=5500  LowerLimit=0
  Subsystem : Subsystem
  Subsystem1 : Subsystem
  Subsystem2 : Subsystem
  Subsystem29 : Subsystem
  Subsystem4 : Subsystem
  Subsystem53 : Subsystem
  Switch{,1..3} (4 alike) : Switch  Criteria=u2 > Threshold
  D1_TEMP : Outport
  D1_LOSS : Outport  Port=2
  D1_LOSS_MEAN : Outport  Port=3
  D1_AVG : Outport  Port=4
  D1_AVG_MEAN : Outport  Port=5
  D1_SW : Outport  Port=6
  D1_SW_MEAN : Outport  Port=7
  D2_TEMP : Outport  Port=8
  D2_LOSS : Outport  Port=9
  D2_LOSS_MEAN : Outport  Port=10
  D2_AVG : Outport  Port=11
  D2_AVG_MEAN : Outport  Port=12
  D2_SW : Outport  Port=13
  D2_SW_MEAN : Outport  Port=14
  wires:
  Mean5/1 -> D2_SW_MEAN/1  "D2_SW_MEAN"
  Subsystem2/1(Out1) -> D2_TEMP/1  "D2_TEMP"
  Mean58/1 -> D1_LOSS_MEAN/1  "D1_LOSS_MEAN"
  PWM1/1 -> Switch2/2
  Mean84/1 -> D1_SW_MEAN/1  "D1_SW_MEAN"
  Saturation1/1 -> Subsystem4/1(In1)
  Subsystem4/1(Out1) -> Add4/2
  Gain3/1 -> Subsystem1/1(In1)
  Mean3/1 -> D2_AVG_MEAN/1  "D2_AVG_MEAN"
  Subsystem1/1(Out1) -> Mean4/1
  Constant6/1 -> Switch3/3
  Constant2/1 -> Switch2/3
  Switch2/1 -> Add34/1
  Constant28/1 -> Switch/3
  Bitwise Operator4/1 -> Logical Operator/2
  Add3/1 -> Mean2/1, D2_LOSS/1  "D2_LOSS"
  Constant3/1 -> Switch2/1
  Constant27/1 -> Relational Operator/2
  Constant7/1 -> Switch3/1
  PWM2/1 -> Switch3/2
  Subsystem/2(Out2) -> Add34/3
  Mean82/1 -> D1_AVG_MEAN/1  "D1_AVG_MEAN"
  Mean4/1 -> Mean5/1, Add3/2, Subsystem2/2(In2), D2_SW/1  "D2_SW"
  Bitwise Operator1/1 -> Logical Operator1/2
  PWM3/1 -> Bitwise Operator4/1, Subsystem29/2(In2)
  Gain6/1 -> Gain3/1, Switch1/1, Relational Operator1/1
  Subsystem29/1(Out1) -> Mean83/1
  Relational Operator1/1 -> Logical Operator1/1
  Relational Operator/1 -> Logical Operator/1
  Switch3/1 -> Add4/1
  Add4/1 -> Subsystem2/1(In1), Add3/1, D2_AVG/1, Mean3/1  "D2_AVG"
  Switch1/1 -> Saturation1/1
  Constant5/1 -> Switch1/3
  Mean83/1 -> Add30/2, Subsystem53/2(In2), D1_SW/1, Mean84/1  "D1_SW"
  Add34/1 -> Mean82/1, D1_AVG/1, Subsystem53/1(In1), Add30/1  "D1_AVG"
  Subsystem53/1(Out1) -> D1_TEMP/1  "D1_TEMP"
  Gain35/1 -> Subsystem29/1(In1)
  Logical Operator/1 -> Switch/2
  Add30/1 -> Mean58/1, D1_LOSS/1  "D1_LOSS"
  Subsystem/1(Out1) -> Add34/2
  Switch/1 -> Saturation11/1
  Constant4/1 -> Relational Operator1/2
  I/1 -> Gain6/1, Gain35/1, Relational Operator/1, Switch/1
  PWM4/1 -> Bitwise Operator1/1, Subsystem1/2(In2)
  Saturation11/1 -> Subsystem/1(In1)
  Mean2/1 -> D2_LOSS_MEAN/1  "D2_LOSS_MEAN"
  Logical Operator1/1 -> Switch1/2
  Subsystem4/2(Out2) -> Add4/3

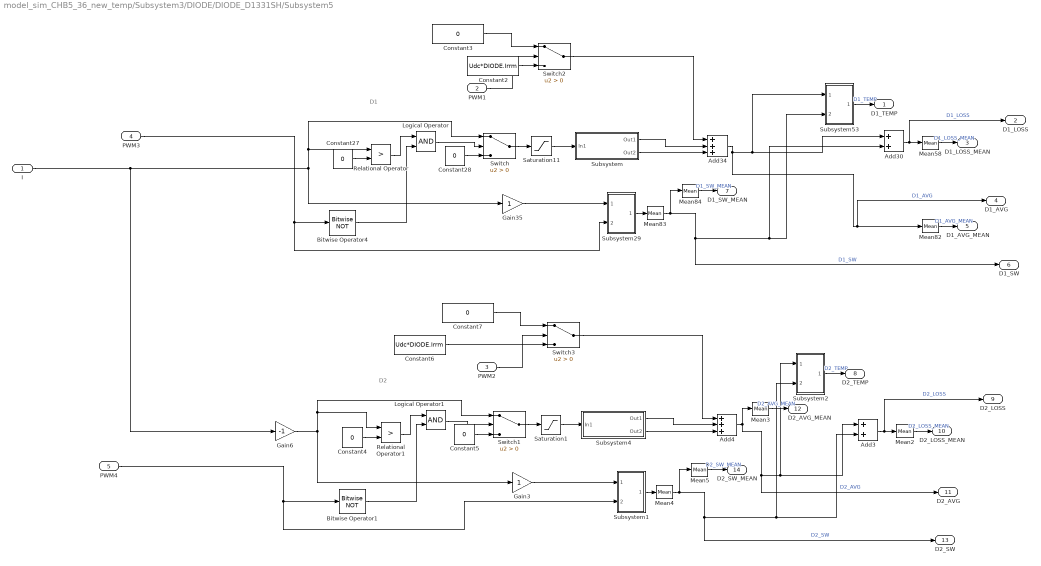
== system model_sim_CHB5_36_new_temp/Subsystem3/DIODE/DIODE_D1331SH/Subsystem5 ==
  note: D1
  note: D2
  I : Inport
  PWM1 : Inport  Port=2
  PWM2 : Inport  Port=3
  PWM3 : Inport  Port=4
  PWM4 : Inport  Port=5
  Add3 : Sum
  Add30 : Sum
  Add34 : Sum  Inputs=+++
  Add4 : Sum  Inputs=+++
  Bitwise Operator1 : simulink/Logic and Bit Operations/Bitwise Operator  logicop=NOT  UseBitMask=off  BitMask=bin2dec('11011001')  BitMaskRealWorld=Stored Integer
  Bitwise Operator4 : simulink/Logic and Bit Operations/Bitwise Operator  logicop=NOT  UseBitMask=off  BitMask=bin2dec('11011001')  BitMaskRealWorld=Stored Integer
  Constant2 : Constant  Value=Udc*DIODE.Irrm
  Constant{3..5,7,27..28} (6 alike) : Constant  Value=0
  Constant6 : Constant  Value=Udc*DIODE.Irrm
  Gain3 : Gain
  Gain35 : Gain
  Gain6 : Gain  Gain=-1
  Logical Operator : Logic  AllPortsSameDT=off  OutDataTypeStr=boolean
  Logical Operator1 : Logic  AllPortsSameDT=off  OutDataTypeStr=boolean
  Mean{2..3,5,58,82,84} (6 alike) : powerlib_meascontrol/Measurements/Mean  Freq=f  Vinit=0  Ts=1e-6
  Mean4 : powerlib_meascontrol/Measurements/Mean  Freq=2000  Vinit=0  Ts=1e-6
  Mean83 : powerlib_meascontrol/Measurements/Mean  Freq=2000  Vinit=0  Ts=1e-6
  Relational Operator : RelationalOperator  Operator=>  OutDataTypeStr=boolean  RndMeth=Simplest
  Relational Operator1 : RelationalOperator  Operator=>  OutDataTypeStr=boolean  RndMeth=Simplest
  Saturation1 : Saturate  UpperLimit=5500  LowerLimit=0
  Saturation11 : Saturate  UpperLimit=5500  LowerLimit=0
  Subsystem : Subsystem
  Subsystem1 : Subsystem
  Subsystem2 : Subsystem
  Subsystem29 : Subsystem
  Subsystem4 : Subsystem
  Subsystem53 : Subsystem
  Switch{,1..3} (4 alike) : Switch  Criteria=u2 > Threshold
  D1_TEMP : Outport
  D1_LOSS : Outport  Port=2
  D1_LOSS_MEAN : Outport  Port=3
  D1_AVG : Outport  Port=4
  D1_AVG_MEAN : Outport  Port=5
  D1_SW : Outport  Port=6
  D1_SW_MEAN : Outport  Port=7
  D2_TEMP : Outport  Port=8
  D2_LOSS : Outport  Port=9
  D2_LOSS_MEAN : Outport  Port=10
  D2_AVG : Outport  Port=11
  D2_AVG_MEAN : Outport  Port=12
  D2_SW : Outport  Port=13
  D2_SW_MEAN : Outport  Port=14
  wires:
  Subsystem4/2(Out2) -> Add4/3
  Logical Operator1/1 -> Switch1/2
  Mean2/1 -> D2_LOSS_MEAN/1  "D2_LOSS_MEAN"
  Saturation11/1 -> Subsystem/1(In1)
  PWM4/1 -> Subsystem1/2(In2), Bitwise Operator1/1
  I/1 -> Switch/1, Relational Operator/1, Gain35/1, Gain6/1
  Constant4/1 -> Relational Operator1/2
  Switch/1 -> Saturation11/1
  Subsystem/1(Out1) -> Add34/2
  Add30/1 -> D1_LOSS/1, Mean58/1  "D1_LOSS"
  Logical Operator/1 -> Switch/2
  Gain35/1 -> Subsystem29/1(In1)
  Subsystem53/1(Out1) -> D1_TEMP/1  "D1_TEMP"
  Add34/1 -> Add30/1, Subsystem53/1(In1), D1_AVG/1, Mean82/1  "D1_AVG"
  Mean83/1 -> Mean84/1, D1_SW/1, Subsystem53/2(In2), Add30/2  "D1_SW"
  Constant5/1 -> Switch1/3
  Switch1/1 -> Saturation1/1
  Add4/1 -> Mean3/1, D2_AVG/1, Add3/1, Subsystem2/1(In1)  "D2_AVG"
  Switch3/1 -> Add4/1
  Relational Operator/1 -> Logical Operator/1
  Relational Operator1/1 -> Logical Operator1/1
  Subsystem29/1(Out1) -> Mean83/1
  Gain6/1 -> Relational Operator1/1, Switch1/1, Gain3/1
  PWM3/1 -> Subsystem29/2(In2), Bitwise Operator4/1
  Bitwise Operator1/1 -> Logical Operator1/2
  Mean4/1 -> D2_SW/1, Subsystem2/2(In2), Add3/2, Mean5/1  "D2_SW"
  Mean82/1 -> D1_AVG_MEAN/1  "D1_AVG_MEAN"
  Subsystem/2(Out2) -> Add34/3
  PWM2/1 -> Switch3/2
  Constant7/1 -> Switch3/1
  Constant27/1 -> Relational Operator/2
  Constant3/1 -> Switch2/1
  Add3/1 -> D2_LOSS/1, Mean2/1  "D2_LOSS"
  Bitwise Operator4/1 -> Logical Operator/2
  Constant28/1 -> Switch/3
  Switch2/1 -> Add34/1
  Constant2/1 -> Switch2/3
  Constant6/1 -> Switch3/3
  Subsystem1/1(Out1) -> Mean4/1
  Mean3/1 -> D2_AVG_MEAN/1  "D2_AVG_MEAN"
  Gain3/1 -> Subsystem1/1(In1)
  Subsystem4/1(Out1) -> Add4/2
  Saturation1/1 -> Subsystem4/1(In1)
  Mean84/1 -> D1_SW_MEAN/1  "D1_SW_MEAN"
  PWM1/1 -> Switch2/2
  Mean58/1 -> D1_LOSS_MEAN/1  "D1_LOSS_MEAN"
  Subsystem2/1(Out1) -> D2_TEMP/1  "D2_TEMP"
  Mean5/1 -> D2_SW_MEAN/1  "D2_SW_MEAN"

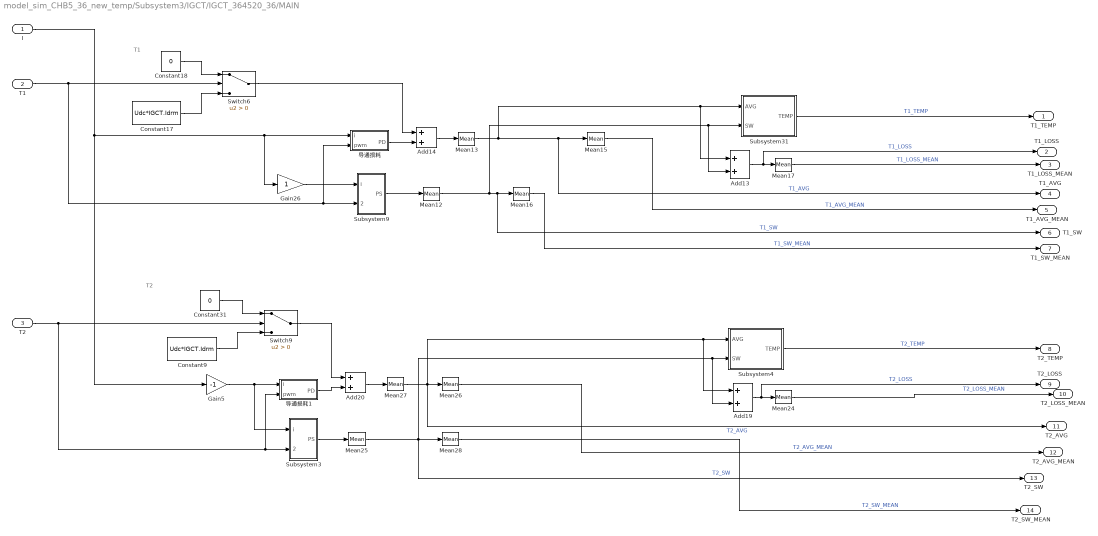
== system model_sim_CHB5_36_new_temp/Subsystem3/IGCT/IGCT_364520_36/MAIN ==
  note: T2
  note: T1
  I : Inport
  T1 : Inport  Port=2
  T2 : Inport  Port=3
  Add{13..14,19..20} (4 alike) : Sum
  Constant17 : Constant  Value=Udc*IGCT.Idrm
  Constant18 : Constant  Value=0
  Constant31 : Constant  Value=0
  Constant9 : Constant  Value=Udc*IGCT.Idrm
  Gain26 : Gain
  Gain5 : Gain  Gain=-1
  Mean{12..13,25,27} (4 alike) : powerlib_meascontrol/Measurements/Mean  Freq=2000  Vinit=0  Ts=1e-6
  Mean{15..16,26,28} (4 alike) : powerlib_meascontrol/Measurements/Mean  Freq=f  Vinit=0  Ts=Ts2
  Mean17 : powerlib_meascontrol/Measurements/Mean  Freq=f  Vinit=0  Ts=1e-6
  Mean24 : powerlib_meascontrol/Measurements/Mean  Freq=f  Vinit=0  Ts=1e-6
  Subsystem3 : Subsystem
  Subsystem31 : Subsystem
  Subsystem4 : Subsystem
  Subsystem9 : Subsystem
  Switch6 : Switch  Criteria=u2 > Threshold
  Switch9 : Switch  Criteria=u2 > Threshold
  导通损耗 : Subsystem
  导通损耗1 : Subsystem
  T1_TEMP : Outport
  T1_LOSS : Outport  Port=2
  T1_LOSS_MEAN : Outport  Port=3
  T1_AVG : Outport  Port=4
  T1_AVG_MEAN : Outport  Port=5
  T1_SW : Outport  Port=6
  T1_SW_MEAN : Outport  Port=7
  T2_TEMP : Outport  Port=8
  T2_LOSS : Outport  Port=9
  T2_LOSS_MEAN : Outport  Port=10
  T2_AVG : Outport  Port=11
  T2_AVG_MEAN : Outport  Port=12
  T2_SW : Outport  Port=13
  T2_SW_MEAN : Outport  Port=14
  wires:
  Mean24/1 -> T2_LOSS_MEAN/1  "T2_LOSS_MEAN"
  Subsystem4/1(TEMP) -> T2_TEMP/1  "T2_TEMP"
  Mean28/1 -> T2_SW_MEAN/1  "T2_SW_MEAN"
  Constant17/1 -> Switch6/3
  Constant18/1 -> Switch6/1
  Subsystem9/1(PS) -> Mean12/1
  Gain26/1 -> Subsystem9/1(i)
  I/1 -> Gain5/1, 导通损耗/1(i), Gain26/1
  导通损耗/1(PD) -> Add14/2
  Switch6/1 -> Add14/1
  导通损耗1/1(PD) -> Add20/2
  Switch9/1 -> Add20/1
  T2/1 -> Switch9/2, Subsystem3/2(pwm), 导通损耗1/2(pwm)
  Add13/1 -> Mean17/1, T1_LOSS/1  "T1_LOSS"
  Mean16/1 -> T1_SW_MEAN/1  "T1_SW_MEAN"
  Subsystem31/1(TEMP) -> T1_TEMP/1  "T1_TEMP"
  Mean26/1 -> T2_AVG_MEAN/1  "T2_AVG_MEAN"
  Add20/1 -> Mean27/1
  Mean17/1 -> T1_LOSS_MEAN/1  "T1_LOSS_MEAN"
  Constant31/1 -> Switch9/1
  Add14/1 -> Mean13/1
  Add19/1 -> Mean24/1, T2_LOSS/1  "T2_LOSS"
  Mean25/1 -> Mean28/1, Subsystem4/2(SW), Add19/2, T2_SW/1  "T2_SW"
  Constant9/1 -> Switch9/3
  Mean12/1 -> Mean16/1, T1_SW/1, Subsystem31/2(SW), Add13/2  "T1_SW"
  Gain5/1 -> 导通损耗1/1(i), Subsystem3/1(i)
  Subsystem3/1(PS) -> Mean25/1
  Mean13/1 -> Subsystem31/1(AVG), Add13/1, Mean15/1, T1_AVG/1  "T1_AVG"
  Mean27/1 -> Subsystem4/1(AVG), Add19/1, Mean26/1, T2_AVG/1  "T2_AVG"
  Mean15/1 -> T1_AVG_MEAN/1  "T1_AVG_MEAN"
  T1/1 -> Switch6/2, Subsystem9/2(pwm), 导通损耗/2(pwm)

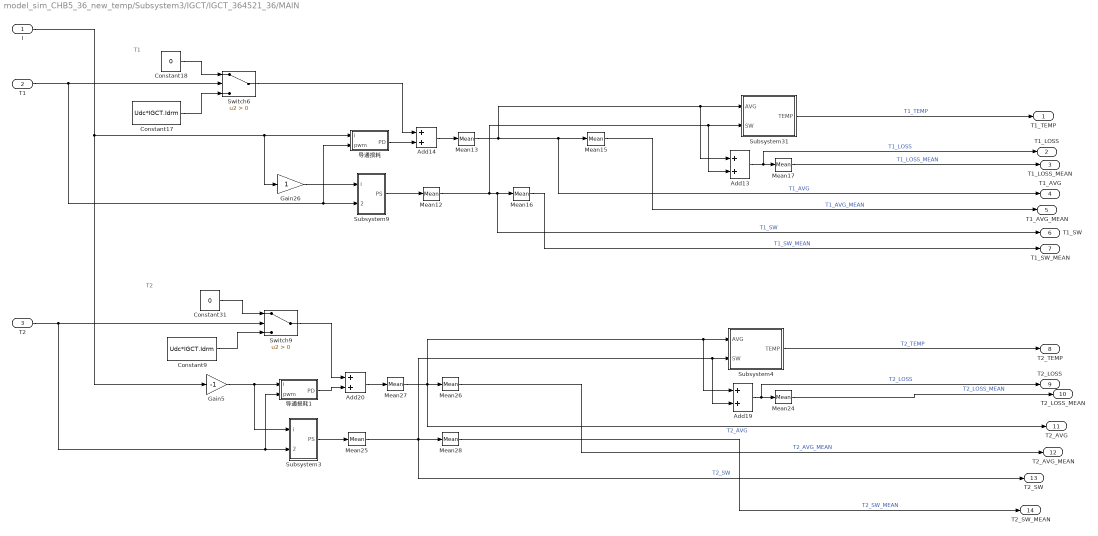
== system model_sim_CHB5_36_new_temp/Subsystem3/IGCT/IGCT_364521_36/MAIN ==
  note: T1
  note: T2
  I : Inport
  T1 : Inport  Port=2
  T2 : Inport  Port=3
  Add{13..14,19..20} (4 alike) : Sum
  Constant17 : Constant  Value=Udc*IGCT.Idrm
  Constant18 : Constant  Value=0
  Constant31 : Constant  Value=0
  Constant9 : Constant  Value=Udc*IGCT.Idrm
  Gain26 : Gain
  Gain5 : Gain  Gain=-1
  Mean{12..13,25,27} (4 alike) : powerlib_meascontrol/Measurements/Mean  Freq=2000  Vinit=0  Ts=1e-6
  Mean{15..16,26,28} (4 alike) : powerlib_meascontrol/Measurements/Mean  Freq=f  Vinit=0  Ts=Ts2
  Mean17 : powerlib_meascontrol/Measurements/Mean  Freq=f  Vinit=0  Ts=1e-6
  Mean24 : powerlib_meascontrol/Measurements/Mean  Freq=f  Vinit=0  Ts=1e-6
  Subsystem3 : Subsystem
  Subsystem31 : Subsystem
  Subsystem4 : Subsystem
  Subsystem9 : Subsystem
  Switch6 : Switch  Criteria=u2 > Threshold
  Switch9 : Switch  Criteria=u2 > Threshold
  导通损耗 : Subsystem
  导通损耗1 : Subsystem
  T1_TEMP : Outport
  T1_LOSS : Outport  Port=2
  T1_LOSS_MEAN : Outport  Port=3
  T1_AVG : Outport  Port=4
  T1_AVG_MEAN : Outport  Port=5
  T1_SW : Outport  Port=6
  T1_SW_MEAN : Outport  Port=7
  T2_TEMP : Outport  Port=8
  T2_LOSS : Outport  Port=9
  T2_LOSS_MEAN : Outport  Port=10
  T2_AVG : Outport  Port=11
  T2_AVG_MEAN : Outport  Port=12
  T2_SW : Outport  Port=13
  T2_SW_MEAN : Outport  Port=14
  wires:
  T1/1 -> 导通损耗/2(pwm), Subsystem9/2(pwm), Switch6/2
  Mean15/1 -> T1_AVG_MEAN/1  "T1_AVG_MEAN"
  Mean27/1 -> T2_AVG/1, Mean26/1, Add19/1, Subsystem4/1(AVG)  "T2_AVG"
  Mean13/1 -> T1_AVG/1, Mean15/1, Add13/1, Subsystem31/1(AVG)  "T1_AVG"
  Subsystem3/1(PS) -> Mean25/1
  Gain5/1 -> Subsystem3/1(i), 导通损耗1/1(i)
  Mean12/1 -> Add13/2, Subsystem31/2(SW), T1_SW/1, Mean16/1  "T1_SW"
  Constant9/1 -> Switch9/3
  Mean25/1 -> T2_SW/1, Add19/2, Subsystem4/2(SW), Mean28/1  "T2_SW"
  Add19/1 -> T2_LOSS/1, Mean24/1  "T2_LOSS"
  Add14/1 -> Mean13/1
  Constant31/1 -> Switch9/1
  Mean17/1 -> T1_LOSS_MEAN/1  "T1_LOSS_MEAN"
  Add20/1 -> Mean27/1
  Mean26/1 -> T2_AVG_MEAN/1  "T2_AVG_MEAN"
  Subsystem31/1(TEMP) -> T1_TEMP/1  "T1_TEMP"
  Mean16/1 -> T1_SW_MEAN/1  "T1_SW_MEAN"
  Add13/1 -> T1_LOSS/1, Mean17/1  "T1_LOSS"
  T2/1 -> 导通损耗1/2(pwm), Subsystem3/2(pwm), Switch9/2
  Switch9/1 -> Add20/1
  导通损耗1/1(PD) -> Add20/2
  Switch6/1 -> Add14/1
  导通损耗/1(PD) -> Add14/2
  I/1 -> Gain26/1, 导通损耗/1(i), Gain5/1
  Gain26/1 -> Subsystem9/1(i)
  Subsystem9/1(PS) -> Mean12/1
  Constant18/1 -> Switch6/1
  Constant17/1 -> Switch6/3
  Mean28/1 -> T2_SW_MEAN/1  "T2_SW_MEAN"
  Subsystem4/1(TEMP) -> T2_TEMP/1  "T2_TEMP"
  Mean24/1 -> T2_LOSS_MEAN/1  "T2_LOSS_MEAN"

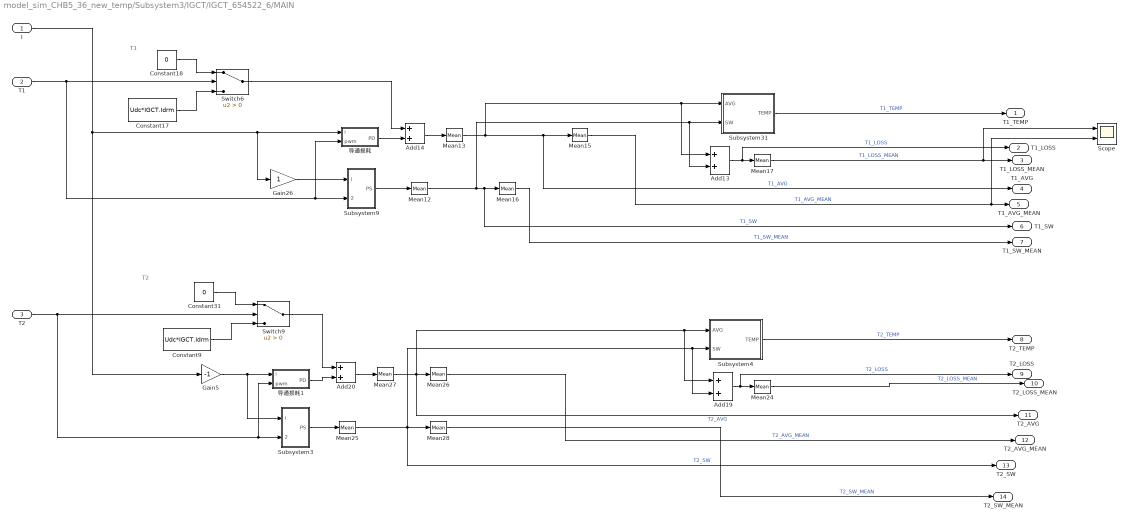
== system model_sim_CHB5_36_new_temp/Subsystem3/IGCT/IGCT_654522_6/MAIN ==
  note: T1
  note: T2
  I : Inport
  T1 : Inport  Port=2
  T2 : Inport  Port=3
  Add{13..14,19..20} (4 alike) : Sum
  Constant17 : Constant  Value=Udc*IGCT.Idrm
  Constant18 : Constant  Value=0
  Constant31 : Constant  Value=0
  Constant9 : Constant  Value=Udc*IGCT.Idrm
  Gain26 : Gain
  Gain5 : Gain  Gain=-1
  Mean{12..13,25,27} (4 alike) : powerlib_meascontrol/Measurements/Mean  Freq=2000  Vinit=0  Ts=1e-6
  Mean{15..16,26,28} (4 alike) : powerlib_meascontrol/Measurements/Mean  Freq=f  Vinit=0  Ts=Ts2
  Mean17 : powerlib_meascontrol/Measurements/Mean  Freq=f  Vinit=0  Ts=1e-6
  Mean24 : powerlib_meascontrol/Measurements/Mean  Freq=f  Vinit=0  Ts=1e-6
  Scope : Scope  NumInputPorts=2
  Subsystem3 : Subsystem
  Subsystem31 : Subsystem
  Subsystem4 : Subsystem
  Subsystem9 : Subsystem
  Switch6 : Switch  Criteria=u2 > Threshold
  Switch9 : Switch  Criteria=u2 > Threshold
  导通损耗 : Subsystem
  导通损耗1 : Subsystem
  T1_TEMP : Outport
  T1_LOSS : Outport  Port=2
  T1_LOSS_MEAN : Outport  Port=3
  T1_AVG : Outport  Port=4
  T1_AVG_MEAN : Outport  Port=5
  T1_SW : Outport  Port=6
  T1_SW_MEAN : Outport  Port=7
  T2_TEMP : Outport  Port=8
  T2_LOSS : Outport  Port=9
  T2_LOSS_MEAN : Outport  Port=10
  T2_AVG : Outport  Port=11
  T2_AVG_MEAN : Outport  Port=12
  T2_SW : Outport  Port=13
  T2_SW_MEAN : Outport  Port=14
  wires:
  T1/1 -> 导通损耗/2(pwm), Subsystem9/2(pwm), Switch6/2
  Mean15/1 -> Scope/2, T1_AVG_MEAN/1  "T1_AVG_MEAN"
  Mean27/1 -> T2_AVG/1, Mean26/1, Add19/1, Subsystem4/1(AVG)  "T2_AVG"
  Mean13/1 -> T1_AVG/1, Mean15/1, Add13/1, Subsystem31/1(AVG)  "T1_AVG"
  Subsystem3/1(PS) -> Mean25/1
  Gain5/1 -> Subsystem3/1(i), 导通损耗1/1(i)
  Mean12/1 -> Add13/2, Subsystem31/2(SW), T1_SW/1, Mean16/1  "T1_SW"
  Constant9/1 -> Switch9/3
  Mean25/1 -> T2_SW/1, Add19/2, Subsystem4/2(SW), Mean28/1  "T2_SW"
  Add19/1 -> T2_LOSS/1, Mean24/1  "T2_LOSS"
  Add14/1 -> Mean13/1
  Constant31/1 -> Switch9/1
  Mean17/1 -> Scope/1, T1_LOSS_MEAN/1  "T1_LOSS_MEAN"
  Add20/1 -> Mean27/1
  Mean26/1 -> T2_AVG_MEAN/1  "T2_AVG_MEAN"
  Subsystem31/1(TEMP) -> T1_TEMP/1  "T1_TEMP"
  Mean16/1 -> T1_SW_MEAN/1  "T1_SW_MEAN"
  Add13/1 -> T1_LOSS/1, Mean17/1  "T1_LOSS"
  T2/1 -> 导通损耗1/2(pwm), Subsystem3/2(pwm), Switch9/2
  Switch9/1 -> Add20/1
  导通损耗1/1(PD) -> Add20/2
  Switch6/1 -> Add14/1
  导通损耗/1(PD) -> Add14/2
  I/1 -> Gain26/1, 导通损耗/1(i), Gain5/1
  Gain26/1 -> Subsystem9/1(i)
  Subsystem9/1(PS) -> Mean12/1
  Constant18/1 -> Switch6/1
  Constant17/1 -> Switch6/3
  Mean28/1 -> T2_SW_MEAN/1  "T2_SW_MEAN"
  Subsystem4/1(TEMP) -> T2_TEMP/1  "T2_TEMP"
  Mean24/1 -> T2_LOSS_MEAN/1  "T2_LOSS_MEAN"

== system model_sim_CHB5_36_new_temp/Subsystem3/DIODE/DIODE_204520/Subsystem5/Subsystem ==
  In1 : Inport
  Gain44 : Gain  Gain=DIODE.rF
  Gain45 : Gain  Gain=DIODE.VF0
  Math Function9 : Math  Operator=magnitude^2  SignedPower=on  SaturateOnIntegerOverflow=on
  Mean79 : powerlib_meascontrol/Measurements/Mean  Freq=2000  Vinit=0  Ts=Ts1
  RMS9 : powerlib_meascontrol/Measurements/RMS  TrueRMS=on  Freq=2000  RMSInit=0  Ts=Ts1
  Out1 : Outport
  Out2 : Outport  Port=2
  wires:
  RMS9/1 -> Math Function9/1
  Gain44/1 -> Out1/1
  Mean79/1 -> Gain45/1
  Math Function9/1 -> Gain44/1
  In1/1 -> Mean79/1, RMS9/1
  Gain45/1 -> Out2/1
